simulink model "SimpleNonLinProb"  (Simulink 7.4)
settings: Solver=ode45  StartTime=0.0  StopTime=10.0  RelTol=1e-3
undefined symbols (not defined in the file or in its folder): magnitude, x1, x2, x3
libraries: BLOM_Lib x8
settings Model: Creator=Kyle  LastModifiedBy=JJK
settings DebuggingCC: StrictBusMsg=ErrorLevel1

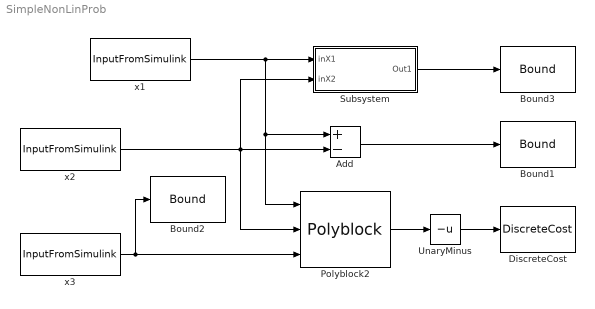
== system SimpleNonLinProb ==
  Add : Sum  Inputs=+-  OutDataType=fixdt(1, 16)  OutScaling=2^-10
  Bound1 : BLOM_Lib/Bound  SystemSampleTime=-1  ub=1  lb=-inf  initial_step=on  intermediate_step=on  final_step=on
  Bound2 : BLOM_Lib/Bound  SystemSampleTime=-1  ub=inf  lb=0  initial_step=on  intermediate_step=on  final_step=on
  Bound3 : BLOM_Lib/Bound  SystemSampleTime=-1  ub=5  lb=-inf  initial_step=on  intermediate_step=on  final_step=on
  DiscreteCost : BLOM_Lib/DiscreteCost  SystemSampleTime=-1  initial_step=on  intermediate_step=on  final_step=on
  Polyblock2 : BLOM_Lib/Polyblock  SystemSampleTime=-1  P=[1 0 0; 0 1 0; 0 0 2; 0 0 1]  K=[3 1 -1 2]  inputs=x1,x2,x3  inputScalar=on  outputScalar=on
  Subsystem : Subsystem
  UnaryMinus : UnaryMinus
  x1 : BLOM_Lib/InputFromSimulink  SystemSampleTime=-1  interpType=Zero-Order Hold  move_blocking_info=[1 0]
  x2 : BLOM_Lib/InputFromSimulink  SystemSampleTime=-1  interpType=Zero-Order Hold  move_blocking_info=[1 0]
  x3 : BLOM_Lib/InputFromSimulink  SystemSampleTime=-1  interpType=Zero-Order Hold  move_blocking_info=[1 0]
  wires:
  x1/1 -> Add/1, Polyblock2/1, Subsystem/1(inX1)
  x2/1 -> Polyblock2/2, Add/2, Subsystem/2(inX2)
  Subsystem/1(Out1) -> Bound3/1
  x3/1 -> Bound2/1, Polyblock2/3
  Polyblock2/1 -> UnaryMinus/1
  UnaryMinus/1 -> DiscreteCost/1
  Add/1 -> Bound1/1

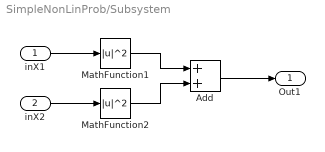
== system SimpleNonLinProb/Subsystem ==
  inX1 : Inport  OutDataType=fixdt(1, 16)  OutScaling=2^0
  inX2 : Inport  Port=2  OutDataType=fixdt(1, 16)  OutScaling=2^0
  Add : Sum  OutDataType=fixdt(1, 16)  OutScaling=2^-10
  MathFunction1 : Math  Operator=magnitude^2  OutDataType=fixdt(1, 16)  OutScaling=2^0  SaturateOnIntegerOverflow=on
  MathFunction2 : Math  Operator=magnitude^2  OutDataType=fixdt(1, 16)  OutScaling=2^0  SaturateOnIntegerOverflow=on
  Out1 : Outport  OutDataType=fixdt(1, 16)  OutScaling=2^0
      mask Display:
      | fprintf(full_name)
      | port_label('input',1,'x1')
      | port_label('input',2,'x2')
      | port_label('input',3,'x3')
  wires:
  inX1/1 -> MathFunction1/1
  inX2/1 -> MathFunction2/1
  Add/1 -> Out1/1
  MathFunction1/1 -> Add/1
  MathFunction2/1 -> Add/2
